simulink model "KR6_dyn_lib"  (R2018a)
settings: Solver=VariableStepAuto  StartTime=0.0  StopTime=10.0  RelTol=1e-3
(part 2 of 2)

== matlab function KR6_dyn_lib/dynamics ==
  data: dq2 input; B output; dq3 input; dq4 input; dq5 input; dq6 input; dq7 input; g input; q2 input; q3 input; q4 input; q5 input; q6 input; Bm output; Phi output; Phim output; G output
function [B,Bm,Phi,Phim,G] = dynamics(dq2,dq3,dq4,dq5,dq6,dq7,g,q2,q3,q4,q5,q6)
%#codegen

%    This function was generated by the Symbolic Math Toolbox version 8.1.
%    27-May-2020 20:53:49

t2 = cos(q2);
t3 = sin(q2);
t4 = sin(q5);
t5 = cos(q3);
t6 = cos(q4);
t7 = sin(q3);
t8 = sin(q4);
t9 = cos(q5);
t10 = cos(q6);
t11 = sin(q6);
t12 = t7.*t8.*1.4164748e7;
t13 = t4.*t5.*t8.*1.79145e5;
t14 = t4.*t6.*t7.*1.79145e5;
t15 = t7.*t8.*t10.*1.42171e5;
t16 = t5.*t8.*t9.*t11.*1.42171e5;
t17 = t6.*t7.*t9.*t11.*1.42171e5;
t18 = t3.*5.02822e-2;
t19 = t3.*t4.*t11.*1.42171e-2;
t20 = t2.*t5.*t8.*1.4164748;
t21 = t2.*t6.*t7.*1.4164748;
t22 = t2.*t7.*t8.*2.37344e-1;
t23 = t2.*t4.*t5.*t6.*1.79145e-2;
t24 = t2.*t5.*t8.*t10.*1.42171e-2;
t25 = t2.*t6.*t7.*t10.*1.42171e-2;
t26 = t2.*t7.*t8.*t9.*4.582e-4;
t27 = t2.*t5.*t6.*t9.*t11.*1.42171e-2;
t28 = t2.*(-6.45733e-1)+t18+t19+t20+t21+t22+t23+t24+t25+t26+t27-t2.*t5.*4.812199-t3.*t4.*4.582e-4-t2.*t7.*6.51847e-2-t3.*t9.*1.79145e-2-t2.*t5.*t6.*2.37344e-1-t2.*t4.*t7.*t8.*1.79145e-2-t2.*t5.*t6.*t9.*4.582e-4-t2.*t7.*t8.*t9.*t11.*1.42171e-2;
t29 = q3.*2.0;
t30 = q5.*2.0;
t31 = cos(t29);
t32 = sin(t29);
t33 = sin(t30);
t34 = cos(t30);
t35 = q6.*2.0;
t36 = cos(t35);
t37 = q4.*2.0;
t38 = cos(t37);
t39 = sin(t37);
t40 = sin(t35);
t41 = t4.*t7.*t8.*1.0579838e-4;
t42 = t5.*t8.*t33.*1.2735850275e-3;
t43 = t6.*t7.*t33.*1.2735850275e-3;
t44 = t7.*t8.*t9.*4.62678618e-3;
t45 = t5.*t8.*t11.*t34.*2.384424e-5;
t46 = t6.*t7.*t11.*t34.*2.384424e-5;
t47 = t4.*t5.*t6.*t40.*4.14863515e-4;
t48 = t5.*t8.*t33.*t36.*2.074317575e-4;
t49 = t6.*t7.*t33.*t36.*2.074317575e-4;
t50 = t4.*t5.*t6.*t11.*5.1892415e-3;
t51 = t7.*t8.*t9.*t10.*2.384424e-5;
t52 = t4.*t5.*t8.*t11.*4.975985e-4;
t53 = t4.*t6.*t7.*t11.*4.975985e-4;
t54 = t10.^2;
t55 = t5.*6.51847e5;
t56 = t7.*4.812199e7;
t68 = t5.*t6.*1.4164748e7;
t69 = t5.*t8.*2.37344e6;
t70 = t6.*t7.*2.37344e6;
t71 = t5.*t6.*t10.*1.42171e5;
t72 = t5.*t8.*t9.*4.582e3;
t73 = t6.*t7.*t9.*4.582e3;
t57 = t12+t13+t14+t15+t16+t17+t55-t56-t68-t69-t70-t71-t72-t73;
t58 = t7.*1.21447802e-2;
t59 = t4.*t7.*t11.*4.4783865e-3;
t74 = t5.*t8.*t34.*1.64952e-6;
t75 = t6.*t7.*t34.*1.64952e-6;
t76 = t5.*t6.*t9.*4.62678618e-3;
t77 = t4.*t5.*t6.*1.0579838e-4;
t78 = t5.*t8.*t9.*6.270075e-4;
t79 = t6.*t7.*t9.*6.270075e-4;
t80 = t4.*t5.*t8.*1.6037e-5;
t81 = t4.*t6.*t7.*1.6037e-5;
t82 = t4.*t7.*t8.*t40.*4.14863515e-4;
t83 = t5.*t6.*t9.*t10.*2.384424e-5;
t84 = t4.*t7.*t8.*t11.*5.1892415e-3;
t60 = t5.*(-3.7807126e-4)+t41+t42+t43+t44+t45+t46+t47+t48+t49+t50+t51+t52+t53+t58+t59-t74-t75-t76-t77-t78-t79-t80-t81-t82-t83-t84-t4.*t7.*1.44333e-4-t7.*t9.*5.6430675e-3;
t61 = t9.^2;
t62 = t6.*7.476336e-2;
t63 = t9.*3.2074e-5;
t64 = t10.*1.0378483e-2;
t65 = t6.*t9.*1.44333e-4;
t66 = t54.*8.2972703e-4;
t67 = t4.*t9.*t11.*4.768848e-5;
t86 = t33.*1.64952e-6;
t87 = t4.*1.254015e-3;
t88 = t9.*t11.*9.95197e-4;
t89 = t61.*2.13230654e-3;
t90 = t54.*t61.*8.2972703e-4;
t85 = t8.*(-4.46189562e-1)+t62+t63+t64+t65+t66+t67-t86-t87-t88-t89-t90-t4.*t6.*5.6430675e-3-t8.*t10.*4.4783865e-3-t6.*t9.*t11.*4.4783865e-3+4.0306203851e-1;
t91 = t9.*4.62678618e-3;
t92 = t4.*1.0579838e-4;
t93 = t9.*t10.*2.384424e-5;
t94 = t9.*1.23472703e-3;
t95 = t9.*t10.*5.1892415e-3;
t96 = t4.*t11.*2.384424e-5;
t97 = t4.*t11.*5.0e-6;
t98 = t2.*t9.*4.582e-4;
t99 = t3.*t5.*t6.*t9.*1.79145e-2;
t100 = t3.*t4.*t5.*t6.*4.582e-4;
t101 = t3.*t4.*t7.*t8.*t11.*1.42171e-2;
t102 = t98+t99+t100+t101-t2.*t4.*1.79145e-2-t2.*t9.*t11.*1.42171e-2-t3.*t4.*t7.*t8.*4.582e-4-t3.*t7.*t8.*t9.*1.79145e-2-t3.*t4.*t5.*t6.*t11.*1.42171e-2;
t103 = t4.*4.478625e-4;
t104 = t4.*t5.*5.6430675e-3;
t105 = t9.*t11.*3.554275e-4;
t106 = t4.*t5.*t6.*6.270075e-4;
t107 = t5.*t8.*t9.*1.0579838e-4;
t108 = t6.*t7.*t9.*1.0579838e-4;
t109 = t5.*t9.*t11.*4.4783865e-3;
t110 = t7.*t8.*t9.*1.6037e-5;
t111 = t5.*t6.*t9.*t11.*4.975985e-4;
t112 = t4.*t8.*t11.*4.4783865e-3;
t114 = t4.*t11.*5.1892415e-3;
t115 = t4.*t10.*t11.*8.2972703e-4;
t113 = t91+t92+t93+t112-t114-t115-t4.*t8.*1.44333e-4-t8.*t9.*5.6430675e-3;
t116 = t3.*t5.*t6.*t9.*t10.*1.42171e-2;
t117 = t116-t2.*t4.*t10.*1.42171e-2-t3.*t5.*t8.*t11.*1.42171e-2-t3.*t6.*t7.*t11.*1.42171e-2-t3.*t7.*t8.*t9.*t10.*1.42171e-2;
t118 = t4.*t10.*3.554275e-4;
t119 = t4.*t5.*t10.*4.4783865e-3;
t120 = t7.*t8.*t10.*2.384424e-5;
t121 = t4.*t5.*t6.*t10.*4.975985e-4;
t122 = t5.*t8.*t9.*t11.*2.384424e-5;
t123 = t6.*t7.*t9.*t11.*2.384424e-5;
t124 = t118+t119+t120+t121+t122+t123-t4.*t5.*t8.*1.23472703e-3-t4.*t6.*t7.*1.23472703e-3-t5.*t6.*t10.*2.384424e-5-t4.*t5.*t8.*t10.*5.1892415e-3-t4.*t6.*t7.*t10.*5.1892415e-3-t4.*t7.*t8.*t10.*4.975985e-4;
t126 = t11.*4.975985e-4;
t125 = t94+t95+t96-t126-t6.*t11.*4.4783865e-3-t8.*t9.*t10.*4.4783865e-3;
t127 = t10.*2.384424e-5;
t128 = q3+q4;
t129 = t10.*5.0e-6;
t130 = sin(t128);
t131 = cos(t128);
t132 = t4.^2;
t133 = t9-t4.*t11;
t134 = t11.^2;
B = reshape([8.714e1,t28,t3.*t57.*(-1.0e-7),t3.*(t12+t13+t14+t15+t16+t17-t68-t69-t70-t71-t72-t73).*(-1.0e-7),t102,t117,0.0,t28,t4.*(-6.270075e-4)+t5.*2.4060995e-1+t7.*3.259235e-3-t8.*4.46189562e-1+t9.*1.6037e-5+t10.*5.1892415e-3+t31.*7.03321055045e-1+t32.*1.00391957e-2+t33.*8.2476e-7+t34.*6.3679251375e-4-t36.*1.0371587875e-4+t62+t65-t4.*t6.*5.6430675e-3+t5.*t6.*1.18672e-2-t5.*t8.*7.082374e-2-t6.*t7.*7.082374e-2-t7.*t8.*1.18672e-2-t8.*t10.*4.4783865e-3-t9.*t11.*4.975985e-4+t6.*t31.*7.476336e-2-t6.*t32.*4.46189562e-1-t8.*t31.*4.46189562e-1-t8.*t32.*7.476336e-2-t11.*t33.*1.192212e-5-t31.*t38.*1.8083421453625e-1-t31.*t39.*4.99715694e-2-t32.*t38.*4.99715694e-2+t34.*t36.*1.0371587875e-4+t32.*t39.*1.8083421453625e-1-t4.*t5.*t6.*8.95725e-4+t4.*t7.*t8.*8.95725e-4+t5.*t6.*t9.*2.291e-5-t5.*t8.*t10.*7.10855e-4-t6.*t7.*t10.*7.10855e-4-t7.*t8.*t9.*2.291e-5-t6.*t9.*t11.*4.4783865e-3-t4.*t6.*t31.*5.6430675e-3+t4.*t8.*t32.*5.6430675e-3+t6.*t9.*t31.*1.44333e-4-t6.*t10.*t32.*4.4783865e-3-t8.*t9.*t32.*1.44333e-4-t8.*t10.*t31.*4.4783865e-3-t4.*t31.*t38.*6.270075e-4+t4.*t31.*t39.*4.62678618e-3+t4.*t32.*t38.*4.62678618e-3+t4.*t32.*t39.*6.270075e-4+t9.*t31.*t38.*1.6037e-5-t9.*t31.*t39.*1.0579838e-4-t9.*t32.*t38.*1.0579838e-4-t10.*t31.*t38.*5.1892415e-3-t9.*t32.*t39.*1.6037e-5-t10.*t31.*t39.*4.975985e-4-t10.*t32.*t38.*4.975985e-4+t10.*t32.*t39.*5.1892415e-3-t31.*t33.*t38.*8.2476e-7-t31.*t34.*t38.*6.3679251375e-4+t32.*t33.*t39.*8.2476e-7-t31.*t36.*t38.*3.1114763625e-4+t32.*t34.*t39.*6.3679251375e-4+t32.*t36.*t39.*3.1114763625e-4-t5.*t6.*t9.*t11.*7.10855e-4+t7.*t8.*t9.*t11.*7.10855e-4-t6.*t9.*t11.*t31.*4.4783865e-3+t8.*t9.*t11.*t32.*4.4783865e-3+t4.*t10.*t31.*t39.*2.384424e-5+t4.*t10.*t32.*t38.*2.384424e-5-t9.*t11.*t31.*t38.*4.975985e-4+t9.*t11.*t31.*t39.*5.1892415e-3+t9.*t11.*t32.*t38.*5.1892415e-3+t9.*t11.*t32.*t39.*4.975985e-4+t11.*t31.*t33.*t38.*1.192212e-5-t11.*t32.*t33.*t39.*1.192212e-5+t9.*t31.*t39.*t40.*4.14863515e-4+t9.*t32.*t38.*t40.*4.14863515e-4-t31.*t34.*t36.*t38.*1.0371587875e-4+t32.*t34.*t36.*t39.*1.0371587875e-4+1.08912681817625,t60,t41+t42+t43+t44+t45+t46+t47+t48+t49+t50+t51+t52+t53-t74-t75-t76-t77-t78-t79-t80-t81-t82-t83-t84,t9.*(-1.1455e-5)+t103+t104+t105+t106+t107+t108+t109+t110+t111-t5.*t6.*1.0581988725e-2-t5.*t9.*1.44333e-4+t7.*t8.*1.0581988725e-2-t4.*t5.*t8.*4.62678618e-3-t4.*t6.*t7.*4.62678618e-3-t4.*t7.*t8.*6.270075e-4-t5.*t6.*t9.*1.6037e-5+t5.*t6.*t36.*4.14863515e-4-t7.*t8.*t36.*4.14863515e-4-t4.*t5.*t8.*t10.*2.384424e-5-t4.*t6.*t7.*t10.*2.384424e-5-t5.*t8.*t9.*t11.*5.1892415e-3-t6.*t7.*t9.*t11.*5.1892415e-3-t7.*t8.*t9.*t11.*4.975985e-4-t5.*t8.*t9.*t40.*4.14863515e-4-t6.*t7.*t9.*t40.*4.14863515e-4,t124,t10.*t131.*(-5.0e-6)+t9.*t11.*t130.*5.0e-6,t3.*t57.*(-1.0e-7),t60,t4.*(-1.254015e-3)+t6.*1.4952672e-1-t8.*8.92379124e-1-t33.*1.64952e-6-t61.*2.13230654e-3+t63+t64+t66+t67-t4.*t6.*1.1286135e-2+t6.*t9.*2.88666e-4-t8.*t10.*8.956773e-3-t9.*t11.*9.95197e-4-t54.*t61.*8.2972703e-4-t6.*t9.*t11.*8.956773e-3+1.84829510642,t85,t113,t125,t97,t3.*(t12+t13+t14+t15+t16+t17-t5.*t6.*1.4164748e7-t5.*t8.*2.37344e6-t6.*t7.*2.37344e6-t5.*t6.*t10.*1.42171e5-t5.*t8.*t9.*4.582e3-t6.*t7.*t9.*4.582e3).*(-1.0e-7),t41+t42+t43+t44+t45+t46+t47+t48+t49+t50+t51+t52+t53-t4.*t5.*t6.*1.0579838e-4-t4.*t5.*t8.*1.6037e-5-t4.*t6.*t7.*1.6037e-5-t5.*t6.*t9.*4.62678618e-3-t5.*t8.*t9.*6.270075e-4-t6.*t7.*t9.*6.270075e-4-t5.*t8.*t34.*1.64952e-6-t6.*t7.*t34.*1.64952e-6-t4.*t7.*t8.*t11.*5.1892415e-3-t5.*t6.*t9.*t10.*2.384424e-5-t4.*t7.*t8.*t40.*4.14863515e-4,t85,t63+t64+t66+t67-t86-t87-t88-t89-t90+4.0306203851e-1,t91+t92+t93-t114-t115,t94+t95+t96-t126,t97,t102,t9.*(-1.1455e-5)+t103+t104+t105+t106+t107+t108+t109+t110+t111-t5.*t6.*1.099685224e-2-t5.*t9.*1.44333e-4+t7.*t8.*1.099685224e-2-t4.*t5.*t8.*4.62678618e-3-t4.*t6.*t7.*4.62678618e-3-t4.*t7.*t8.*6.270075e-4-t5.*t6.*t9.*1.6037e-5+t5.*t6.*t54.*8.2972703e-4-t7.*t8.*t54.*8.2972703e-4-t4.*t5.*t8.*t10.*2.384424e-5-t4.*t6.*t7.*t10.*2.384424e-5-t5.*t8.*t9.*t11.*5.1892415e-3-t6.*t7.*t9.*t11.*5.1892415e-3-t7.*t8.*t9.*t11.*4.975985e-4-t5.*t8.*t9.*t10.*t11.*8.2972703e-4-t6.*t7.*t9.*t10.*t11.*8.2972703e-4,t113,t91+t92+t93-t4.*t11.*5.1892415e-3-t4.*t10.*t11.*8.2972703e-4,t134.*8.2972703e-4+1.016712521e-2,t127,t129,t117,t124,t125,t11.*(-4.975985e-4)+t94+t95+t96,t127,1.23472703e-3,0.0,0.0,-t5.*(t6.*t10.*5.0e-6-t8.*t9.*t11.*5.0e-6)+t7.*(t8.*t10.*5.0e-6+t6.*t9.*t11.*5.0e-6),t97,t97,t129,0.0,5.0e-6],[7,7]);
if nargout > 1
    Bm = reshape([2.1e1./1.0e1,0.0,0.0,0.0,0.0,0.0,0.0,0.0,2.1e1./1.0e1,t2.*(-2.1e1./1.0e3),0.0,t8.*t130.*(2.1e1./1.0e3),t9.*t131.*(2.1e1./1.0e3)-t33.*t130.*1.05e-2,t11.*(t11.*t131.*(2.1e1./1.0e3)+t9.*t10.*t130.*(2.1e1./1.0e3))+t4.*t10.*t130.*(2.1e1./1.0e3),0.0,t2.*(-2.1e1./1.0e3),2.1e1./1.0e1,2.1e1./1.0e3,t6.*(-2.1e1./1.0e3),t132.*(-2.1e1./1.0e3),t10.*t133.*(-2.1e1./1.0e3),0.0,0.0,2.1e1./1.0e3,2.1e1./1.0e1,t6.*(-2.1e1./1.0e3),t132.*(-2.1e1./1.0e3),t10.*t133.*(-2.1e1./1.0e3),0.0,0.0,0.0,t6.*(-2.1e1./1.0e3),2.1e1./1.0e1,t9.*(-2.1e1./1.0e3),t134.*(-2.1e1./1.0e3),0.0,0.0,0.0,0.0,t9.*(-2.1e1./1.0e3),2.1e1./1.0e1,t10.*(-2.1e1./1.0e3),0.0,0.0,0.0,0.0,0.0,t10.*(-2.1e1./1.0e3),2.1e1./1.0e1],[7,7]);
end
if nargout > 2
    t135 = dq2.^2;
    t136 = dq5.^2;
    t137 = dq3.^2;
    t138 = dq4.^2;
    t139 = dq6.^2;
    t140 = t9.*t136.*1.0579838e-4;
    t141 = dq3.*dq5.*t33.*2.547170055e-3;
    t142 = dq4.*dq5.*t33.*2.547170055e-3;
    t143 = t31.*t38.*t135.*4.99715694e-2;
    t144 = t5.*t6.*t135.*3.541187e-2;
    t145 = t5.*t8.*t135.*5.9336e-3;
    t146 = t6.*t7.*t135.*5.9336e-3;
    t147 = t4.*t10.*t139.*2.384424e-5;
    t148 = dq3.*dq5.*t11.*t34.*4.768848e-5;
    t149 = dq3.*dq6.*t10.*t33.*2.384424e-5;
    t150 = dq4.*dq5.*t11.*t34.*4.768848e-5;
    t151 = dq4.*dq6.*t10.*t33.*2.384424e-5;
    t152 = t9.*t31.*t38.*t135.*1.0579838e-4;
    t153 = t10.*t31.*t38.*t135.*4.975985e-4;
    t154 = t9.*t31.*t39.*t135.*1.6037e-5;
    t155 = t9.*t32.*t38.*t135.*1.6037e-5;
    t156 = t4.*t32.*t39.*t135.*4.62678618e-3;
    t157 = dq3.*dq5.*t33.*t36.*4.14863515e-4;
    t158 = dq3.*dq6.*t34.*t40.*4.14863515e-4;
    t159 = dq4.*dq5.*t33.*t36.*4.14863515e-4;
    t160 = dq4.*dq6.*t34.*t40.*4.14863515e-4;
    t161 = t5.*t6.*t10.*t135.*3.554275e-4;
    t162 = t5.*t8.*t9.*t135.*1.1455e-5;
    t163 = t6.*t7.*t9.*t135.*1.1455e-5;
    t164 = dq5.*dq7.*t9.*t11.*5.0e-6;
    t165 = dq6.*dq7.*t4.*t10.*5.0e-6;
    t166 = dq3.*dq5.*t4.*t11.*9.95197e-4;
    t167 = dq4.*dq5.*t4.*t11.*9.95197e-4;
    t168 = dq2.*dq5.*t5.*t8.*t34.*2.547170055e-3;
    t169 = dq2.*dq5.*t6.*t7.*t34.*2.547170055e-3;
    t170 = dq2.*dq5.*t5.*t8.*t36.*4.14863515e-4;
    t171 = dq2.*dq5.*t6.*t7.*t36.*4.14863515e-4;
    t172 = dq2.*dq5.*t5.*t8.*t33.*3.29904e-6;
    t173 = dq2.*dq5.*t6.*t7.*t33.*3.29904e-6;
    t174 = t9.*t11.*t32.*t39.*t135.*5.1892415e-3;
    t175 = t4.*t10.*t32.*t39.*t135.*2.384424e-5;
    t176 = dq2.*dq5.*t4.*t5.*t6.*9.25357236e-3;
    t177 = dq2.*dq6.*t4.*t5.*t6.*1.23472703e-3;
    t178 = t11.*t31.*t33.*t39.*t135.*1.192212e-5;
    t179 = t11.*t32.*t33.*t38.*t135.*1.192212e-5;
    t180 = t9.*t32.*t39.*t40.*t135.*4.14863515e-4;
    t181 = dq2.*dq5.*t4.*t5.*t8.*1.254015e-3;
    t182 = dq2.*dq5.*t4.*t6.*t7.*1.254015e-3;
    t183 = dq2.*dq5.*t7.*t8.*t9.*2.1159676e-4;
    t184 = dq2.*dq5.*t5.*t8.*t34.*t36.*4.14863515e-4;
    t185 = dq2.*dq5.*t6.*t7.*t34.*t36.*4.14863515e-4;
    t186 = dq2.*dq5.*t5.*t6.*t9.*t11.*1.0378483e-2;
    t187 = dq2.*dq5.*t4.*t5.*t6.*t10.*4.768848e-5;
    t188 = dq2.*dq6.*t4.*t5.*t6.*t10.*1.0378483e-2;
    t189 = dq2.*dq5.*t5.*t8.*t9.*t11.*9.95197e-4;
    t190 = dq2.*dq5.*t6.*t7.*t9.*t11.*9.95197e-4;
    t191 = dq2.*dq6.*t4.*t5.*t8.*t10.*9.95197e-4;
    t192 = dq2.*dq6.*t4.*t6.*t7.*t10.*9.95197e-4;
    t193 = dq2.*dq7.*t7.*t8.*t9.*t11.*5.0e-6;
    t194 = dq2.*dq5.*t5.*t6.*t9.*t40.*8.2972703e-4;
    t195 = dq2.*dq6.*t5.*t8.*t10.*t34.*2.384424e-5;
    t196 = dq2.*dq6.*t6.*t7.*t10.*t34.*2.384424e-5;
    t197 = dq2.*dq6.*t4.*t5.*t6.*t36.*8.2972703e-4;
    Phi = [t2.*t135.*5.02822e-2+t3.*t135.*6.45733e-1-t2.*t4.*t135.*4.582e-4-t2.*t4.*t136.*4.582e-4+t3.*t5.*t135.*4.812199+t3.*t5.*t137.*4.812199+t3.*t7.*t135.*6.51847e-2-t2.*t9.*t135.*1.79145e-2-t2.*t9.*t136.*1.79145e-2+t3.*t7.*t137.*6.51847e-2-dq2.*dq3.*t2.*t5.*1.303694e-1+dq2.*dq3.*t2.*t7.*9.624398+dq2.*dq5.*t3.*t4.*3.5829e-2-dq2.*dq5.*t3.*t9.*9.164e-4+t3.*t5.*t6.*t135.*2.37344e-1+t3.*t5.*t6.*t137.*2.37344e-1-t3.*t5.*t8.*t135.*1.4164748-t3.*t6.*t7.*t135.*1.4164748+t2.*t4.*t11.*t135.*1.42171e-2+t3.*t5.*t6.*t138.*2.37344e-1+t2.*t4.*t11.*t136.*1.42171e-2-t3.*t5.*t8.*t137.*1.4164748-t3.*t6.*t7.*t137.*1.4164748-t3.*t7.*t8.*t135.*2.37344e-1-t3.*t5.*t8.*t138.*1.4164748-t3.*t6.*t7.*t138.*1.4164748-t3.*t7.*t8.*t137.*2.37344e-1+t2.*t4.*t11.*t139.*1.42171e-2-t3.*t7.*t8.*t138.*2.37344e-1+dq2.*dq3.*t2.*t5.*t6.*2.8329496+dq2.*dq4.*t2.*t5.*t6.*2.8329496+dq2.*dq3.*t2.*t5.*t8.*4.74688e-1+dq2.*dq3.*t2.*t6.*t7.*4.74688e-1+dq2.*dq4.*t2.*t5.*t8.*4.74688e-1+dq2.*dq4.*t2.*t6.*t7.*4.74688e-1+dq3.*dq4.*t3.*t5.*t6.*4.74688e-1-dq2.*dq3.*t2.*t7.*t8.*2.8329496-dq2.*dq4.*t2.*t7.*t8.*2.8329496-dq3.*dq4.*t3.*t5.*t8.*2.8329496-dq3.*dq4.*t3.*t6.*t7.*2.8329496+dq2.*dq6.*t3.*t4.*t10.*2.84342e-2-dq3.*dq4.*t3.*t7.*t8.*4.74688e-1+dq2.*dq5.*t3.*t9.*t11.*2.84342e-2-dq5.*dq6.*t2.*t9.*t10.*2.84342e-2-t3.*t4.*t5.*t6.*t135.*1.79145e-2-t3.*t4.*t5.*t6.*t136.*1.79145e-2-t3.*t4.*t5.*t6.*t137.*1.79145e-2-t3.*t4.*t5.*t6.*t138.*1.79145e-2+t3.*t4.*t7.*t8.*t135.*1.79145e-2+t3.*t4.*t7.*t8.*t136.*1.79145e-2+t3.*t5.*t6.*t9.*t135.*4.582e-4+t3.*t4.*t7.*t8.*t137.*1.79145e-2+t3.*t5.*t6.*t9.*t136.*4.582e-4+t3.*t4.*t7.*t8.*t138.*1.79145e-2+t3.*t5.*t6.*t9.*t137.*4.582e-4+t3.*t5.*t6.*t9.*t138.*4.582e-4-t3.*t5.*t8.*t10.*t135.*1.42171e-2-t3.*t6.*t7.*t10.*t135.*1.42171e-2-t3.*t7.*t8.*t9.*t135.*4.582e-4-t3.*t5.*t8.*t10.*t137.*1.42171e-2-t3.*t6.*t7.*t10.*t137.*1.42171e-2-t3.*t7.*t8.*t9.*t136.*4.582e-4-t3.*t5.*t8.*t10.*t138.*1.42171e-2-t3.*t6.*t7.*t10.*t138.*1.42171e-2-t3.*t7.*t8.*t9.*t137.*4.582e-4-t3.*t5.*t8.*t10.*t139.*1.42171e-2-t3.*t6.*t7.*t10.*t139.*1.42171e-2-t3.*t7.*t8.*t9.*t138.*4.582e-4-t3.*t5.*t6.*t9.*t11.*t135.*1.42171e-2-t3.*t5.*t6.*t9.*t11.*t136.*1.42171e-2-t3.*t5.*t6.*t9.*t11.*t137.*1.42171e-2-t3.*t5.*t6.*t9.*t11.*t138.*1.42171e-2-t3.*t5.*t6.*t9.*t11.*t139.*1.42171e-2+t3.*t7.*t8.*t9.*t11.*t135.*1.42171e-2+t3.*t7.*t8.*t9.*t11.*t136.*1.42171e-2+t3.*t7.*t8.*t9.*t11.*t137.*1.42171e-2+t3.*t7.*t8.*t9.*t11.*t138.*1.42171e-2+t3.*t7.*t8.*t9.*t11.*t139.*1.42171e-2-dq2.*dq3.*t2.*t4.*t5.*t8.*3.5829e-2-dq2.*dq3.*t2.*t4.*t6.*t7.*3.5829e-2+dq2.*dq5.*t2.*t4.*t5.*t6.*9.164e-4-dq2.*dq4.*t2.*t4.*t5.*t8.*3.5829e-2-dq2.*dq4.*t2.*t4.*t6.*t7.*3.5829e-2-dq3.*dq4.*t3.*t4.*t5.*t6.*3.5829e-2+dq2.*dq3.*t2.*t5.*t6.*t10.*2.84342e-2-dq2.*dq5.*t2.*t4.*t7.*t8.*9.164e-4-dq3.*dq5.*t3.*t4.*t5.*t8.*9.164e-4-dq3.*dq5.*t3.*t4.*t6.*t7.*9.164e-4+dq2.*dq3.*t2.*t5.*t8.*t9.*9.164e-4+dq2.*dq3.*t2.*t6.*t7.*t9.*9.164e-4+dq2.*dq4.*t2.*t5.*t6.*t10.*2.84342e-2+dq2.*dq5.*t2.*t5.*t6.*t9.*3.5829e-2+dq3.*dq4.*t3.*t4.*t7.*t8.*3.5829e-2-dq4.*dq5.*t3.*t4.*t5.*t8.*9.164e-4-dq4.*dq5.*t3.*t4.*t6.*t7.*9.164e-4+dq2.*dq4.*t2.*t5.*t8.*t9.*9.164e-4+dq2.*dq4.*t2.*t6.*t7.*t9.*9.164e-4+dq3.*dq4.*t3.*t5.*t6.*t9.*9.164e-4-dq2.*dq3.*t2.*t7.*t8.*t10.*2.84342e-2-dq2.*dq4.*t2.*t7.*t8.*t10.*2.84342e-2-dq2.*dq5.*t2.*t7.*t8.*t9.*3.5829e-2-dq3.*dq4.*t3.*t5.*t8.*t10.*2.84342e-2-dq3.*dq4.*t3.*t6.*t7.*t10.*2.84342e-2-dq3.*dq5.*t3.*t5.*t8.*t9.*3.5829e-2-dq3.*dq5.*t3.*t6.*t7.*t9.*3.5829e-2-dq2.*dq6.*t2.*t5.*t8.*t11.*2.84342e-2-dq2.*dq6.*t2.*t6.*t7.*t11.*2.84342e-2-dq3.*dq4.*t3.*t7.*t8.*t9.*9.164e-4-dq3.*dq6.*t3.*t5.*t6.*t11.*2.84342e-2-dq4.*dq5.*t3.*t5.*t8.*t9.*3.5829e-2-dq4.*dq5.*t3.*t6.*t7.*t9.*3.5829e-2-dq4.*dq6.*t3.*t5.*t6.*t11.*2.84342e-2+dq3.*dq6.*t3.*t7.*t8.*t11.*2.84342e-2+dq4.*dq6.*t3.*t7.*t8.*t11.*2.84342e-2-dq2.*dq5.*t2.*t4.*t5.*t6.*t11.*2.84342e-2+dq2.*dq5.*t2.*t4.*t7.*t8.*t11.*2.84342e-2+dq3.*dq5.*t3.*t4.*t5.*t8.*t11.*2.84342e-2+dq3.*dq5.*t3.*t4.*t6.*t7.*t11.*2.84342e-2-dq5.*dq6.*t3.*t4.*t5.*t6.*t10.*2.84342e-2-dq2.*dq3.*t2.*t5.*t8.*t9.*t11.*2.84342e-2-dq2.*dq3.*t2.*t6.*t7.*t9.*t11.*2.84342e-2+dq2.*dq6.*t2.*t5.*t6.*t9.*t10.*2.84342e-2+dq4.*dq5.*t3.*t4.*t5.*t8.*t11.*2.84342e-2+dq4.*dq5.*t3.*t4.*t6.*t7.*t11.*2.84342e-2-dq2.*dq4.*t2.*t5.*t8.*t9.*t11.*2.84342e-2-dq2.*dq4.*t2.*t6.*t7.*t9.*t11.*2.84342e-2-dq3.*dq4.*t3.*t5.*t6.*t9.*t11.*2.84342e-2+dq5.*dq6.*t3.*t4.*t7.*t8.*t10.*2.84342e-2-dq2.*dq6.*t2.*t7.*t8.*t9.*t10.*2.84342e-2-dq3.*dq6.*t3.*t5.*t8.*t9.*t10.*2.84342e-2-dq3.*dq6.*t3.*t6.*t7.*t9.*t10.*2.84342e-2+dq3.*dq4.*t3.*t7.*t8.*t9.*t11.*2.84342e-2-dq4.*dq6.*t3.*t5.*t8.*t9.*t10.*2.84342e-2-dq4.*dq6.*t3.*t6.*t7.*t9.*t10.*2.84342e-2;t4.*t136.*1.1455e-5+t5.*t137.*1.21447802e-2+t7.*t137.*3.7807126e-4+t9.*t136.*4.478625e-4+dq2.*dq3.*t5.*3.259235e-3-dq2.*dq5.*t4.*1.6037e-5-dq2.*dq3.*t7.*2.4060995e-1-dq2.*dq4.*t6.*4.46189562e-1-dq2.*dq4.*t8.*7.476336e-2-dq2.*dq5.*t9.*6.270075e-4-dq2.*dq6.*t11.*5.1892415e-3+dq2.*dq3.*t31.*2.00783914e-2-dq2.*dq3.*t32.*1.40664211009-dq2.*dq5.*t33.*1.2735850275e-3+dq2.*dq5.*t34.*1.64952e-6+dq2.*dq6.*t40.*2.074317575e-4+t4.*t5.*t136.*1.44333e-4-t4.*t5.*t137.*1.44333e-4+t5.*t9.*t136.*5.6430675e-3-t4.*t11.*t136.*3.554275e-4-t5.*t9.*t137.*5.6430675e-3-t4.*t11.*t139.*3.554275e-4-dq2.*dq3.*t5.*t6.*7.082374e-2-dq2.*dq4.*t5.*t6.*7.082374e-2-dq2.*dq5.*t4.*t6.*1.44333e-4-dq2.*dq3.*t5.*t8.*1.18672e-2-dq2.*dq3.*t6.*t7.*1.18672e-2+dq2.*dq4.*t4.*t8.*5.6430675e-3-dq2.*dq4.*t5.*t8.*1.18672e-2-dq2.*dq4.*t6.*t7.*1.18672e-2+dq2.*dq3.*t7.*t8.*7.082374e-2+dq2.*dq4.*t7.*t8.*7.082374e-2+dq3.*dq5.*t5.*t8.*1.0581988725e-2+dq3.*dq5.*t6.*t7.*1.0581988725e-2-dq2.*dq4.*t6.*t10.*4.4783865e-3+dq2.*dq5.*t4.*t11.*4.975985e-4-dq2.*dq5.*t6.*t9.*5.6430675e-3+dq4.*dq5.*t5.*t8.*1.0581988725e-2+dq4.*dq5.*t6.*t7.*1.0581988725e-2-dq2.*dq4.*t8.*t9.*1.44333e-4+dq2.*dq6.*t8.*t11.*4.4783865e-3-dq2.*dq6.*t9.*t10.*4.975985e-4+dq5.*dq6.*t9.*t10.*7.10855e-4-dq2.*dq3.*t6.*t31.*8.92379124e-1-dq2.*dq3.*t6.*t32.*1.4952672e-1-dq2.*dq4.*t6.*t31.*4.46189562e-1-dq2.*dq3.*t8.*t31.*1.4952672e-1-dq2.*dq4.*t6.*t32.*7.476336e-2+dq2.*dq3.*t8.*t32.*8.92379124e-1-dq2.*dq4.*t8.*t31.*7.476336e-2+dq2.*dq4.*t8.*t32.*4.46189562e-1-dq2.*dq6.*t10.*t33.*1.192212e-5-dq2.*dq5.*t11.*t34.*2.384424e-5-dq2.*dq3.*t31.*t38.*9.99431388e-2+dq2.*dq3.*t31.*t39.*3.616684290725e-1+dq2.*dq3.*t32.*t38.*3.616684290725e-1-dq2.*dq4.*t31.*t38.*9.99431388e-2+dq2.*dq3.*t32.*t39.*9.99431388e-2+dq2.*dq4.*t31.*t39.*3.616684290725e-1+dq2.*dq4.*t32.*t38.*3.616684290725e-1-dq2.*dq5.*t33.*t36.*2.074317575e-4+dq2.*dq4.*t32.*t39.*9.99431388e-2-dq2.*dq6.*t34.*t40.*2.074317575e-4+t4.*t5.*t6.*t136.*1.6037e-5-t4.*t5.*t6.*t137.*1.6037e-5-t4.*t5.*t6.*t138.*1.6037e-5-t4.*t5.*t8.*t136.*1.0579838e-4-t4.*t6.*t7.*t136.*1.0579838e-4+t4.*t5.*t8.*t137.*1.0579838e-4+t4.*t6.*t7.*t137.*1.0579838e-4+t4.*t5.*t8.*t138.*1.0579838e-4+t4.*t6.*t7.*t138.*1.0579838e-4-t4.*t7.*t8.*t136.*1.6037e-5-t4.*t5.*t11.*t136.*4.4783865e-3+t4.*t7.*t8.*t137.*1.6037e-5+t5.*t6.*t9.*t136.*6.270075e-4+t4.*t5.*t11.*t137.*4.4783865e-3+t4.*t7.*t8.*t138.*1.6037e-5-t5.*t6.*t9.*t137.*6.270075e-4-t5.*t6.*t9.*t138.*6.270075e-4-t5.*t8.*t9.*t136.*4.62678618e-3-t6.*t7.*t9.*t136.*4.62678618e-3-t4.*t5.*t11.*t139.*4.4783865e-3+t5.*t8.*t9.*t137.*4.62678618e-3+t6.*t7.*t9.*t137.*4.62678618e-3+t5.*t8.*t9.*t138.*4.62678618e-3+t6.*t7.*t9.*t138.*4.62678618e-3-t7.*t8.*t9.*t136.*6.270075e-4+t5.*t6.*t11.*t139.*2.384424e-5+t7.*t8.*t9.*t137.*6.270075e-4+t7.*t8.*t9.*t138.*6.270075e-4-t7.*t8.*t11.*t139.*2.384424e-5+t5.*t6.*t33.*t137.*1.2735850275e-3+t5.*t6.*t33.*t138.*1.2735850275e-3-t5.*t6.*t34.*t137.*1.64952e-6-t5.*t6.*t34.*t138.*1.64952e-6-t7.*t8.*t33.*t137.*1.2735850275e-3-t7.*t8.*t33.*t138.*1.2735850275e-3+t7.*t8.*t34.*t137.*1.64952e-6+t7.*t8.*t34.*t138.*1.64952e-6+dq2.*dq3.*t4.*t5.*t8.*8.95725e-4+dq2.*dq3.*t4.*t6.*t7.*8.95725e-4-dq2.*dq5.*t4.*t5.*t6.*2.291e-5-dq3.*dq4.*t4.*t5.*t6.*3.2074e-5+dq2.*dq4.*t4.*t5.*t8.*8.95725e-4+dq2.*dq4.*t4.*t6.*t7.*8.95725e-4+dq3.*dq4.*t4.*t5.*t8.*2.1159676e-4+dq3.*dq4.*t4.*t6.*t7.*2.1159676e-4-dq3.*dq6.*t4.*t5.*t6.*1.23472703e-3-dq4.*dq6.*t4.*t5.*t6.*1.23472703e-3-dq2.*dq3.*t5.*t6.*t10.*7.10855e-4+dq2.*dq5.*t4.*t7.*t8.*2.291e-5+dq3.*dq4.*t4.*t7.*t8.*3.2074e-5-dq2.*dq3.*t5.*t8.*t9.*2.291e-5-dq2.*dq3.*t6.*t7.*t9.*2.291e-5-dq2.*dq4.*t5.*t6.*t10.*7.10855e-4-dq2.*dq5.*t5.*t6.*t9.*8.95725e-4-dq3.*dq4.*t5.*t6.*t9.*1.254015e-3-dq2.*dq4.*t5.*t8.*t9.*2.291e-5-dq2.*dq4.*t6.*t7.*t9.*2.291e-5+dq2.*dq5.*t4.*t6.*t11.*4.4783865e-3+dq3.*dq6.*t4.*t7.*t8.*1.23472703e-3+dq3.*dq4.*t5.*t8.*t9.*9.25357236e-3+dq3.*dq4.*t6.*t7.*t9.*9.25357236e-3+dq4.*dq6.*t4.*t7.*t8.*1.23472703e-3+dq2.*dq3.*t7.*t8.*t10.*7.10855e-4+dq2.*dq4.*t7.*t8.*t10.*7.10855e-4+dq2.*dq5.*t7.*t8.*t9.*8.95725e-4+dq3.*dq4.*t7.*t8.*t9.*1.254015e-3+dq2.*dq6.*t5.*t8.*t11.*7.10855e-4+dq2.*dq6.*t6.*t7.*t11.*7.10855e-4+dq3.*dq6.*t5.*t8.*t10.*2.384424e-5+dq3.*dq6.*t6.*t7.*t10.*2.384424e-5-dq2.*dq6.*t6.*t9.*t10.*4.4783865e-3+dq3.*dq7.*t5.*t8.*t10.*5.0e-6+dq3.*dq7.*t6.*t7.*t10.*5.0e-6+dq4.*dq6.*t5.*t8.*t10.*2.384424e-5+dq4.*dq6.*t6.*t7.*t10.*2.384424e-5-dq5.*dq6.*t5.*t8.*t9.*1.23472703e-3-dq5.*dq6.*t6.*t7.*t9.*1.23472703e-3+dq2.*dq4.*t8.*t9.*t11.*4.4783865e-3+dq4.*dq7.*t5.*t8.*t10.*5.0e-6+dq4.*dq7.*t6.*t7.*t10.*5.0e-6+dq5.*dq6.*t5.*t9.*t10.*8.956773e-3+dq6.*dq7.*t5.*t6.*t11.*5.0e-6-dq6.*dq7.*t7.*t8.*t11.*5.0e-6+dq2.*dq3.*t4.*t6.*t32.*1.1286135e-2+dq2.*dq3.*t4.*t8.*t31.*1.1286135e-2+dq2.*dq4.*t4.*t6.*t32.*5.6430675e-3-dq2.*dq5.*t4.*t6.*t31.*1.44333e-4+dq2.*dq4.*t4.*t8.*t31.*5.6430675e-3+dq2.*dq5.*t4.*t8.*t32.*1.44333e-4+dq3.*dq4.*t5.*t6.*t33.*2.547170055e-3-dq2.*dq3.*t6.*t9.*t32.*2.88666e-4-dq2.*dq3.*t6.*t10.*t31.*8.956773e-3-dq3.*dq4.*t5.*t6.*t34.*3.29904e-6-dq2.*dq3.*t8.*t9.*t31.*2.88666e-4-dq2.*dq4.*t6.*t9.*t32.*1.44333e-4-dq2.*dq4.*t6.*t10.*t31.*4.4783865e-3-dq2.*dq5.*t6.*t9.*t31.*5.6430675e-3-dq2.*dq4.*t8.*t9.*t31.*1.44333e-4+dq3.*dq5.*t5.*t8.*t33.*3.29904e-6+dq3.*dq5.*t6.*t7.*t33.*3.29904e-6+dq2.*dq3.*t8.*t10.*t32.*8.956773e-3-dq3.*dq4.*t7.*t8.*t33.*2.547170055e-3+dq3.*dq5.*t5.*t8.*t34.*2.547170055e-3+dq3.*dq5.*t6.*t7.*t34.*2.547170055e-3+dq4.*dq5.*t5.*t8.*t33.*3.29904e-6+dq4.*dq5.*t6.*t7.*t33.*3.29904e-6+dq2.*dq4.*t8.*t10.*t32.*4.4783865e-3+dq2.*dq5.*t8.*t9.*t32.*5.6430675e-3+dq3.*dq4.*t7.*t8.*t34.*3.29904e-6+dq4.*dq5.*t5.*t8.*t34.*2.547170055e-3+dq4.*dq5.*t6.*t7.*t34.*2.547170055e-3+dq2.*dq6.*t6.*t11.*t32.*4.4783865e-3-dq3.*dq5.*t5.*t8.*t36.*4.14863515e-4-dq3.*dq5.*t6.*t7.*t36.*4.14863515e-4+dq2.*dq6.*t8.*t11.*t31.*4.4783865e-3-dq4.*dq5.*t5.*t8.*t36.*4.14863515e-4-dq4.*dq5.*t6.*t7.*t36.*4.14863515e-4-dq5.*dq6.*t5.*t6.*t40.*8.2972703e-4+dq5.*dq6.*t7.*t8.*t40.*8.2972703e-4+dq2.*dq3.*t4.*t31.*t38.*9.25357236e-3+dq2.*dq3.*t4.*t31.*t39.*1.254015e-3+dq2.*dq3.*t4.*t32.*t38.*1.254015e-3+dq2.*dq4.*t4.*t31.*t38.*9.25357236e-3-dq2.*dq3.*t4.*t32.*t39.*9.25357236e-3+dq2.*dq4.*t4.*t31.*t39.*1.254015e-3+dq2.*dq4.*t4.*t32.*t38.*1.254015e-3-dq2.*dq5.*t4.*t31.*t38.*1.6037e-5-dq2.*dq4.*t4.*t32.*t39.*9.25357236e-3+dq2.*dq5.*t4.*t31.*t39.*1.0579838e-4+dq2.*dq5.*t4.*t32.*t38.*1.0579838e-4+dq2.*dq5.*t4.*t32.*t39.*1.6037e-5-dq2.*dq3.*t9.*t31.*t38.*2.1159676e-4-dq2.*dq3.*t9.*t31.*t39.*3.2074e-5-dq2.*dq3.*t9.*t32.*t38.*3.2074e-5-dq2.*dq3.*t10.*t31.*t38.*9.95197e-4-dq2.*dq4.*t9.*t31.*t38.*2.1159676e-4+dq2.*dq3.*t9.*t32.*t39.*2.1159676e-4+dq2.*dq3.*t10.*t31.*t39.*1.0378483e-2+dq2.*dq3.*t10.*t32.*t38.*1.0378483e-2-dq2.*dq4.*t9.*t31.*t39.*3.2074e-5-dq2.*dq4.*t9.*t32.*t38.*3.2074e-5-dq2.*dq4.*t10.*t31.*t38.*9.95197e-4-dq2.*dq5.*t9.*t31.*t38.*6.270075e-4+dq2.*dq3.*t10.*t32.*t39.*9.95197e-4+dq2.*dq4.*t9.*t32.*t39.*2.1159676e-4+dq2.*dq4.*t10.*t31.*t39.*1.0378483e-2+dq2.*dq4.*t10.*t32.*t38.*1.0378483e-2+dq2.*dq5.*t9.*t31.*t39.*4.62678618e-3+dq2.*dq5.*t9.*t32.*t38.*4.62678618e-3+dq2.*dq4.*t10.*t32.*t39.*9.95197e-4+dq2.*dq5.*t9.*t32.*t39.*6.270075e-4+dq2.*dq6.*t11.*t31.*t38.*5.1892415e-3+dq2.*dq6.*t11.*t31.*t39.*4.975985e-4+dq2.*dq6.*t11.*t32.*t38.*4.975985e-4-dq2.*dq6.*t11.*t32.*t39.*5.1892415e-3+dq2.*dq3.*t31.*t33.*t39.*1.64952e-6+dq2.*dq3.*t32.*t33.*t38.*1.64952e-6+dq2.*dq3.*t31.*t34.*t39.*1.2735850275e-3+dq2.*dq3.*t32.*t34.*t38.*1.2735850275e-3+dq2.*dq4.*t31.*t33.*t39.*1.64952e-6+dq2.*dq4.*t32.*t33.*t38.*1.64952e-6+dq2.*dq5.*t31.*t33.*t38.*1.2735850275e-3+dq2.*dq4.*t31.*t34.*t39.*1.2735850275e-3+dq2.*dq4.*t32.*t34.*t38.*1.2735850275e-3-dq2.*dq5.*t31.*t34.*t38.*1.64952e-6+dq2.*dq3.*t31.*t36.*t39.*6.222952725e-4+dq2.*dq3.*t32.*t36.*t38.*6.222952725e-4-dq2.*dq5.*t32.*t33.*t39.*1.2735850275e-3+dq2.*dq4.*t31.*t36.*t39.*6.222952725e-4+dq2.*dq4.*t32.*t36.*t38.*6.222952725e-4+dq2.*dq5.*t32.*t34.*t39.*1.64952e-6+dq2.*dq6.*t31.*t38.*t40.*6.222952725e-4-dq2.*dq6.*t32.*t39.*t40.*6.222952725e-4-t4.*t5.*t6.*t11.*t136.*4.975985e-4+t4.*t5.*t6.*t11.*t137.*4.975985e-4+t4.*t5.*t6.*t11.*t138.*4.975985e-4+t4.*t5.*t8.*t11.*t136.*5.1892415e-3+t4.*t6.*t7.*t11.*t136.*5.1892415e-3-t4.*t5.*t6.*t11.*t139.*4.975985e-4-t4.*t5.*t8.*t11.*t137.*5.1892415e-3-t4.*t6.*t7.*t11.*t137.*5.1892415e-3-t4.*t5.*t8.*t11.*t138.*5.1892415e-3-t4.*t6.*t7.*t11.*t138.*5.1892415e-3+t4.*t7.*t8.*t11.*t136.*4.975985e-4+t4.*t5.*t8.*t11.*t139.*5.1892415e-3+t4.*t6.*t7.*t11.*t139.*5.1892415e-3-t4.*t7.*t8.*t11.*t137.*4.975985e-4-t4.*t7.*t8.*t11.*t138.*4.975985e-4-t5.*t8.*t9.*t10.*t136.*2.384424e-5-t6.*t7.*t9.*t10.*t136.*2.384424e-5+t4.*t7.*t8.*t11.*t139.*4.975985e-4+t5.*t8.*t9.*t10.*t137.*2.384424e-5+t6.*t7.*t9.*t10.*t137.*2.384424e-5+t5.*t8.*t9.*t10.*t138.*2.384424e-5+t6.*t7.*t9.*t10.*t138.*2.384424e-5+t5.*t8.*t9.*t10.*t139.*2.384424e-5+t6.*t7.*t9.*t10.*t139.*2.384424e-5+t4.*t5.*t8.*t40.*t136.*4.14863515e-4+t4.*t6.*t7.*t40.*t136.*4.14863515e-4+t5.*t6.*t11.*t34.*t137.*2.384424e-5-t4.*t5.*t8.*t40.*t137.*4.14863515e-4-t4.*t6.*t7.*t40.*t137.*4.14863515e-4+t5.*t6.*t11.*t34.*t138.*2.384424e-5-t4.*t5.*t8.*t40.*t138.*4.14863515e-4-t4.*t6.*t7.*t40.*t138.*4.14863515e-4-t7.*t8.*t11.*t34.*t137.*2.384424e-5-t7.*t8.*t11.*t34.*t138.*2.384424e-5+t5.*t6.*t33.*t36.*t137.*2.074317575e-4+t5.*t6.*t33.*t36.*t138.*2.074317575e-4-t7.*t8.*t33.*t36.*t137.*2.074317575e-4-t7.*t8.*t33.*t36.*t138.*2.074317575e-4+dq2.*dq5.*t4.*t5.*t6.*t11.*7.10855e-4+dq3.*dq4.*t4.*t5.*t6.*t11.*9.95197e-4-dq3.*dq4.*t4.*t5.*t8.*t11.*1.0378483e-2-dq3.*dq4.*t4.*t6.*t7.*t11.*1.0378483e-2-dq2.*dq5.*t4.*t7.*t8.*t11.*7.10855e-4-dq3.*dq4.*t4.*t7.*t8.*t11.*9.95197e-4+dq2.*dq3.*t5.*t8.*t9.*t11.*7.10855e-4+dq2.*dq3.*t6.*t7.*t9.*t11.*7.10855e-4-dq2.*dq6.*t5.*t6.*t9.*t10.*7.10855e-4+dq2.*dq4.*t5.*t8.*t9.*t11.*7.10855e-4+dq2.*dq4.*t6.*t7.*t9.*t11.*7.10855e-4+dq3.*dq4.*t5.*t8.*t9.*t10.*4.768848e-5+dq3.*dq4.*t6.*t7.*t9.*t10.*4.768848e-5+dq3.*dq6.*t5.*t6.*t9.*t11.*4.768848e-5-dq5.*dq7.*t4.*t5.*t8.*t11.*5.0e-6-dq5.*dq7.*t4.*t6.*t7.*t11.*5.0e-6+dq3.*dq7.*t5.*t6.*t9.*t11.*5.0e-6+dq4.*dq6.*t5.*t6.*t9.*t11.*4.768848e-5+dq5.*dq6.*t5.*t6.*t9.*t10.*9.95197e-4+dq2.*dq6.*t7.*t8.*t9.*t10.*7.10855e-4+dq4.*dq7.*t5.*t6.*t9.*t11.*5.0e-6-dq5.*dq6.*t5.*t8.*t9.*t10.*1.0378483e-2-dq5.*dq6.*t6.*t7.*t9.*t10.*1.0378483e-2-dq3.*dq6.*t7.*t8.*t9.*t11.*4.768848e-5-dq3.*dq7.*t7.*t8.*t9.*t11.*5.0e-6-dq4.*dq6.*t7.*t8.*t9.*t11.*4.768848e-5-dq5.*dq6.*t7.*t8.*t9.*t10.*9.95197e-4+dq6.*dq7.*t5.*t8.*t9.*t10.*5.0e-6+dq6.*dq7.*t6.*t7.*t9.*t10.*5.0e-6-dq4.*dq7.*t7.*t8.*t9.*t11.*5.0e-6+dq2.*dq5.*t4.*t6.*t11.*t31.*4.4783865e-3+dq3.*dq6.*t4.*t5.*t6.*t36.*8.2972703e-4+dq4.*dq6.*t4.*t5.*t6.*t36.*8.2972703e-4-dq2.*dq5.*t4.*t8.*t11.*t32.*4.4783865e-3+dq2.*dq3.*t6.*t9.*t11.*t32.*8.956773e-3+dq3.*dq4.*t5.*t6.*t11.*t34.*4.768848e-5+dq2.*dq3.*t8.*t9.*t11.*t31.*8.956773e-3+dq2.*dq4.*t6.*t9.*t11.*t32.*4.4783865e-3-dq2.*dq6.*t6.*t9.*t10.*t31.*4.4783865e-3-dq3.*dq4.*t4.*t5.*t8.*t40.*8.2972703e-4-dq3.*dq4.*t4.*t6.*t7.*t40.*8.2972703e-4-dq3.*dq6.*t4.*t7.*t8.*t36.*8.2972703e-4+dq2.*dq4.*t8.*t9.*t11.*t31.*4.4783865e-3-dq3.*dq5.*t5.*t8.*t11.*t33.*4.768848e-5-dq3.*dq5.*t6.*t7.*t11.*t33.*4.768848e-5-dq4.*dq6.*t4.*t7.*t8.*t36.*8.2972703e-4+dq3.*dq6.*t5.*t8.*t10.*t34.*2.384424e-5+dq3.*dq6.*t6.*t7.*t10.*t34.*2.384424e-5-dq4.*dq5.*t5.*t8.*t11.*t33.*4.768848e-5-dq4.*dq5.*t6.*t7.*t11.*t33.*4.768848e-5+dq2.*dq6.*t8.*t9.*t10.*t32.*4.4783865e-3-dq3.*dq4.*t7.*t8.*t11.*t34.*4.768848e-5+dq4.*dq6.*t5.*t8.*t10.*t34.*2.384424e-5+dq4.*dq6.*t6.*t7.*t10.*t34.*2.384424e-5-dq5.*dq6.*t5.*t8.*t9.*t36.*8.2972703e-4-dq5.*dq6.*t6.*t7.*t9.*t36.*8.2972703e-4+dq3.*dq4.*t5.*t6.*t33.*t36.*4.14863515e-4+dq2.*dq3.*t4.*t10.*t31.*t38.*4.768848e-5+dq2.*dq4.*t4.*t10.*t31.*t38.*4.768848e-5-dq2.*dq3.*t4.*t10.*t32.*t39.*4.768848e-5-dq2.*dq4.*t4.*t10.*t32.*t39.*4.768848e-5+dq2.*dq5.*t4.*t11.*t31.*t38.*4.975985e-4-dq3.*dq4.*t7.*t8.*t33.*t36.*4.14863515e-4+dq3.*dq5.*t5.*t8.*t34.*t36.*4.14863515e-4+dq3.*dq5.*t6.*t7.*t34.*t36.*4.14863515e-4-dq2.*dq5.*t4.*t11.*t31.*t39.*5.1892415e-3-dq2.*dq5.*t4.*t11.*t32.*t38.*5.1892415e-3+dq4.*dq5.*t5.*t8.*t34.*t36.*4.14863515e-4+dq4.*dq5.*t6.*t7.*t34.*t36.*4.14863515e-4-dq2.*dq5.*t4.*t11.*t32.*t39.*4.975985e-4-dq2.*dq6.*t4.*t11.*t31.*t39.*2.384424e-5-dq2.*dq6.*t4.*t11.*t32.*t38.*2.384424e-5+dq2.*dq3.*t9.*t11.*t31.*t38.*1.0378483e-2+dq2.*dq3.*t9.*t11.*t31.*t39.*9.95197e-4+dq2.*dq3.*t9.*t11.*t32.*t38.*9.95197e-4+dq2.*dq4.*t9.*t11.*t31.*t38.*1.0378483e-2-dq3.*dq6.*t5.*t8.*t33.*t40.*4.14863515e-4-dq3.*dq6.*t6.*t7.*t33.*t40.*4.14863515e-4-dq2.*dq3.*t9.*t11.*t32.*t39.*1.0378483e-2+dq2.*dq4.*t9.*t11.*t31.*t39.*9.95197e-4+dq2.*dq4.*t9.*t11.*t32.*t38.*9.95197e-4+dq2.*dq5.*t9.*t10.*t31.*t39.*2.384424e-5+dq2.*dq5.*t9.*t10.*t32.*t38.*2.384424e-5-dq2.*dq6.*t9.*t10.*t31.*t38.*4.975985e-4-dq4.*dq6.*t5.*t8.*t33.*t40.*4.14863515e-4-dq4.*dq6.*t6.*t7.*t33.*t40.*4.14863515e-4-dq2.*dq4.*t9.*t11.*t32.*t39.*1.0378483e-2+dq2.*dq6.*t9.*t10.*t31.*t39.*5.1892415e-3+dq2.*dq6.*t9.*t10.*t32.*t38.*5.1892415e-3+dq2.*dq6.*t9.*t10.*t32.*t39.*4.975985e-4-dq2.*dq3.*t11.*t31.*t33.*t39.*2.384424e-5-dq2.*dq3.*t11.*t32.*t33.*t38.*2.384424e-5-dq2.*dq4.*t11.*t31.*t33.*t39.*2.384424e-5-dq2.*dq4.*t11.*t32.*t33.*t38.*2.384424e-5+dq2.*dq6.*t10.*t31.*t33.*t38.*1.192212e-5-dq2.*dq5.*t4.*t31.*t39.*t40.*4.14863515e-4-dq2.*dq5.*t4.*t32.*t38.*t40.*4.14863515e-4+dq2.*dq5.*t11.*t31.*t34.*t38.*2.384424e-5-dq2.*dq6.*t10.*t32.*t33.*t39.*1.192212e-5+dq2.*dq3.*t9.*t31.*t38.*t40.*8.2972703e-4-dq2.*dq5.*t11.*t32.*t34.*t39.*2.384424e-5+dq2.*dq6.*t9.*t31.*t36.*t39.*8.2972703e-4+dq2.*dq6.*t9.*t32.*t36.*t38.*8.2972703e-4+dq2.*dq4.*t9.*t31.*t38.*t40.*8.2972703e-4-dq2.*dq3.*t9.*t32.*t39.*t40.*8.2972703e-4-dq2.*dq4.*t9.*t32.*t39.*t40.*8.2972703e-4+dq2.*dq3.*t31.*t34.*t36.*t39.*2.074317575e-4+dq2.*dq3.*t32.*t34.*t36.*t38.*2.074317575e-4+dq2.*dq5.*t31.*t33.*t36.*t38.*2.074317575e-4+dq2.*dq4.*t31.*t34.*t36.*t39.*2.074317575e-4+dq2.*dq4.*t32.*t34.*t36.*t38.*2.074317575e-4-dq2.*dq5.*t32.*t33.*t36.*t39.*2.074317575e-4+dq2.*dq6.*t31.*t34.*t38.*t40.*2.074317575e-4-dq2.*dq6.*t32.*t34.*t39.*t40.*2.074317575e-4;t140+t141+t142+t143+t144+t145+t146+t147+t148+t149+t150+t151+t152+t153+t154+t155+t156+t157+t158+t159+t160+t161+t162+t163+t164+t165+t166+t167+t168+t169+t170+t171+t172+t173+t174+t175+t176+t177+t178+t179+t180+t181+t182+t183+t184+t185+t186+t187+t188+t189+t190+t191+t192+t193+t194+t195+t196+t197-t4.*t136.*4.62678618e-3-t5.*t135.*1.6296175e-3+t7.*t135.*1.20304975e-1-t6.*t138.*4.46189562e-1-t8.*t138.*7.476336e-2-t10.*t139.*4.975985e-4-t31.*t135.*1.00391957e-2+t32.*t135.*7.03321055045e-1-dq3.*dq5.*t4.*3.2074e-5-dq3.*dq4.*t6.*8.92379124e-1-dq4.*dq5.*t4.*3.2074e-5-dq3.*dq4.*t8.*1.4952672e-1-dq5.*dq6.*t4.*1.23472703e-3-dq3.*dq5.*t9.*1.254015e-3-dq4.*dq5.*t9.*1.254015e-3-dq3.*dq6.*t11.*1.0378483e-2-dq4.*dq6.*t11.*1.0378483e-2-dq3.*dq5.*t34.*3.29904e-6-dq4.*dq5.*t34.*3.29904e-6-dq3.*dq6.*t40.*4.14863515e-4-dq4.*dq6.*t40.*4.14863515e-4+t4.*t8.*t136.*5.6430675e-3+t4.*t8.*t138.*5.6430675e-3-t4.*t10.*t136.*2.384424e-5-t7.*t8.*t135.*3.541187e-2-t8.*t9.*t136.*1.44333e-4-t6.*t10.*t138.*4.4783865e-3-t6.*t10.*t139.*4.4783865e-3-t8.*t9.*t138.*1.44333e-4-t9.*t11.*t136.*5.1892415e-3-t9.*t11.*t139.*5.1892415e-3+t6.*t31.*t135.*4.46189562e-1+t6.*t32.*t135.*7.476336e-2+t8.*t31.*t135.*7.476336e-2-t8.*t32.*t135.*4.46189562e-1-t9.*t40.*t136.*4.14863515e-4-t31.*t39.*t135.*1.8083421453625e-1-t32.*t38.*t135.*1.8083421453625e-1-t32.*t39.*t135.*4.99715694e-2+dq2.*dq5.*t4.*t7.*1.1286135e-2-dq3.*dq5.*t4.*t6.*2.88666e-4+dq3.*dq4.*t4.*t8.*1.1286135e-2-dq4.*dq5.*t4.*t6.*2.88666e-4-dq2.*dq5.*t5.*t8.*1.0581988725e-2-dq2.*dq5.*t6.*t7.*1.0581988725e-2-dq2.*dq5.*t7.*t9.*2.88666e-4-dq3.*dq4.*t6.*t10.*8.956773e-3-dq3.*dq5.*t6.*t9.*1.1286135e-2-dq3.*dq4.*t8.*t9.*2.88666e-4-dq4.*dq5.*t6.*t9.*1.1286135e-2-dq5.*dq6.*t4.*t10.*1.0378483e-2+dq3.*dq6.*t8.*t11.*8.956773e-3-dq3.*dq6.*t9.*t10.*9.95197e-4+dq4.*dq6.*t8.*t11.*8.956773e-3-dq4.*dq6.*t9.*t10.*9.95197e-4-dq5.*dq6.*t4.*t36.*8.2972703e-4-t4.*t5.*t8.*t135.*4.478625e-4-t4.*t6.*t7.*t135.*4.478625e-4-t7.*t8.*t10.*t135.*3.554275e-4+t8.*t9.*t11.*t136.*4.4783865e-3+t8.*t9.*t11.*t138.*4.4783865e-3+t8.*t9.*t11.*t139.*4.4783865e-3-t4.*t6.*t32.*t135.*5.6430675e-3-t4.*t8.*t31.*t135.*5.6430675e-3+t6.*t9.*t32.*t135.*1.44333e-4+t6.*t10.*t31.*t135.*4.4783865e-3+t8.*t9.*t31.*t135.*1.44333e-4-t8.*t10.*t32.*t135.*4.4783865e-3-t4.*t31.*t38.*t135.*4.62678618e-3-t4.*t31.*t39.*t135.*6.270075e-4-t4.*t32.*t38.*t135.*6.270075e-4-t9.*t32.*t39.*t135.*1.0579838e-4-t10.*t31.*t39.*t135.*5.1892415e-3-t10.*t32.*t38.*t135.*5.1892415e-3-t10.*t32.*t39.*t135.*4.975985e-4-t31.*t33.*t39.*t135.*8.2476e-7-t32.*t33.*t38.*t135.*8.2476e-7-t31.*t34.*t39.*t135.*6.3679251375e-4-t32.*t34.*t38.*t135.*6.3679251375e-4-t31.*t36.*t39.*t135.*3.1114763625e-4-t32.*t36.*t38.*t135.*3.1114763625e-4-dq2.*dq5.*t4.*t7.*t8.*9.25357236e-3-dq2.*dq5.*t5.*t6.*t9.*2.1159676e-4-dq2.*dq6.*t4.*t7.*t8.*1.23472703e-3-dq2.*dq5.*t5.*t8.*t9.*3.2074e-5-dq2.*dq5.*t6.*t7.*t9.*3.2074e-5+dq2.*dq6.*t4.*t7.*t10.*8.956773e-3+dq3.*dq5.*t4.*t6.*t11.*8.956773e-3+dq4.*dq5.*t4.*t6.*t11.*8.956773e-3-dq2.*dq6.*t5.*t8.*t10.*2.384424e-5-dq2.*dq6.*t6.*t7.*t10.*2.384424e-5-dq2.*dq7.*t5.*t8.*t10.*5.0e-6-dq2.*dq7.*t6.*t7.*t10.*5.0e-6+dq5.*dq6.*t4.*t8.*t10.*8.956773e-3+dq2.*dq5.*t7.*t9.*t11.*8.956773e-3-dq3.*dq6.*t6.*t9.*t10.*8.956773e-3+dq3.*dq4.*t8.*t9.*t11.*8.956773e-3-dq4.*dq6.*t6.*t9.*t10.*8.956773e-3-t5.*t8.*t9.*t11.*t135.*3.554275e-4-t6.*t7.*t9.*t11.*t135.*3.554275e-4-t6.*t9.*t11.*t32.*t135.*4.4783865e-3-t8.*t9.*t11.*t31.*t135.*4.4783865e-3-t4.*t10.*t31.*t38.*t135.*2.384424e-5-t9.*t11.*t31.*t38.*t135.*5.1892415e-3-t9.*t11.*t31.*t39.*t135.*4.975985e-4-t9.*t11.*t32.*t38.*t135.*4.975985e-4-t9.*t31.*t38.*t40.*t135.*4.14863515e-4-t31.*t34.*t36.*t39.*t135.*1.0371587875e-4-t32.*t34.*t36.*t38.*t135.*1.0371587875e-4-dq2.*dq5.*t4.*t7.*t8.*t10.*4.768848e-5-dq2.*dq6.*t4.*t7.*t8.*t10.*1.0378483e-2-dq2.*dq7.*t5.*t6.*t9.*t11.*5.0e-6-dq2.*dq5.*t7.*t8.*t9.*t11.*1.0378483e-2-dq2.*dq6.*t4.*t7.*t8.*t36.*8.2972703e-4-dq2.*dq5.*t5.*t8.*t11.*t33.*4.768848e-5-dq2.*dq5.*t6.*t7.*t11.*t33.*4.768848e-5-dq2.*dq5.*t7.*t8.*t9.*t40.*8.2972703e-4-dq2.*dq6.*t5.*t8.*t33.*t40.*4.14863515e-4-dq2.*dq6.*t6.*t7.*t33.*t40.*4.14863515e-4;t140+t141+t142+t143+t144+t145+t146+t147+t148+t149+t150+t151+t152+t153+t154+t155+t156+t157+t158+t159+t160+t161+t162+t163+t164+t165+t166+t167+t168+t169+t170+t171+t172+t173+t174+t175+t176+t177+t178+t179+t180+t181+t182+t183+t184+t185+t186+t187+t188+t189+t190+t191+t192+t193+t194+t195+t196+t197-t4.*t136.*4.62678618e-3+t6.*t135.*2.23094781e-1+t6.*t137.*4.46189562e-1+t8.*t135.*3.738168e-2+t8.*t137.*7.476336e-2-t10.*t139.*4.975985e-4-dq3.*dq5.*t4.*3.2074e-5-dq4.*dq5.*t4.*3.2074e-5-dq5.*dq6.*t4.*1.23472703e-3-dq3.*dq5.*t9.*1.254015e-3-dq4.*dq5.*t9.*1.254015e-3-dq3.*dq6.*t11.*1.0378483e-2-dq4.*dq6.*t11.*1.0378483e-2-dq3.*dq5.*t34.*3.29904e-6-dq4.*dq5.*t34.*3.29904e-6-dq3.*dq6.*t40.*4.14863515e-4-dq4.*dq6.*t40.*4.14863515e-4-t4.*t8.*t135.*2.82153375e-3-t4.*t8.*t137.*5.6430675e-3-t4.*t10.*t136.*2.384424e-5-t7.*t8.*t135.*3.541187e-2+t6.*t10.*t135.*2.23919325e-3+t8.*t9.*t135.*7.21665e-5+t6.*t10.*t137.*4.4783865e-3+t8.*t9.*t137.*1.44333e-4-t9.*t11.*t136.*5.1892415e-3-t9.*t11.*t139.*5.1892415e-3+t6.*t31.*t135.*2.23094781e-1+t6.*t32.*t135.*3.738168e-2+t8.*t31.*t135.*3.738168e-2-t8.*t32.*t135.*2.23094781e-1-t9.*t40.*t136.*4.14863515e-4-t31.*t39.*t135.*1.8083421453625e-1-t32.*t38.*t135.*1.8083421453625e-1-t32.*t39.*t135.*4.99715694e-2-dq2.*dq5.*t5.*t8.*1.0581988725e-2-dq2.*dq5.*t6.*t7.*1.0581988725e-2-dq5.*dq6.*t4.*t10.*1.0378483e-2-dq3.*dq6.*t9.*t10.*9.95197e-4-dq4.*dq6.*t9.*t10.*9.95197e-4-dq5.*dq6.*t4.*t36.*8.2972703e-4-t4.*t5.*t8.*t135.*4.478625e-4-t4.*t6.*t7.*t135.*4.478625e-4-t7.*t8.*t10.*t135.*3.554275e-4-t8.*t9.*t11.*t135.*2.23919325e-3-t8.*t9.*t11.*t137.*4.4783865e-3-t4.*t6.*t32.*t135.*2.82153375e-3-t4.*t8.*t31.*t135.*2.82153375e-3+t6.*t9.*t32.*t135.*7.21665e-5+t6.*t10.*t31.*t135.*2.23919325e-3+t8.*t9.*t31.*t135.*7.21665e-5-t8.*t10.*t32.*t135.*2.23919325e-3-t4.*t31.*t38.*t135.*4.62678618e-3-t4.*t31.*t39.*t135.*6.270075e-4-t4.*t32.*t38.*t135.*6.270075e-4-t9.*t32.*t39.*t135.*1.0579838e-4-t10.*t31.*t39.*t135.*5.1892415e-3-t10.*t32.*t38.*t135.*5.1892415e-3-t10.*t32.*t39.*t135.*4.975985e-4-t31.*t33.*t39.*t135.*8.2476e-7-t32.*t33.*t38.*t135.*8.2476e-7-t31.*t34.*t39.*t135.*6.3679251375e-4-t32.*t34.*t38.*t135.*6.3679251375e-4-t31.*t36.*t39.*t135.*3.1114763625e-4-t32.*t36.*t38.*t135.*3.1114763625e-4-dq2.*dq5.*t4.*t7.*t8.*9.25357236e-3-dq2.*dq5.*t5.*t6.*t9.*2.1159676e-4-dq2.*dq6.*t4.*t7.*t8.*1.23472703e-3-dq2.*dq5.*t5.*t8.*t9.*3.2074e-5-dq2.*dq5.*t6.*t7.*t9.*3.2074e-5-dq2.*dq6.*t5.*t8.*t10.*2.384424e-5-dq2.*dq6.*t6.*t7.*t10.*2.384424e-5-dq2.*dq7.*t5.*t8.*t10.*5.0e-6-dq2.*dq7.*t6.*t7.*t10.*5.0e-6-t5.*t8.*t9.*t11.*t135.*3.554275e-4-t6.*t7.*t9.*t11.*t135.*3.554275e-4-t6.*t9.*t11.*t32.*t135.*2.23919325e-3-t8.*t9.*t11.*t31.*t135.*2.23919325e-3-t4.*t10.*t31.*t38.*t135.*2.384424e-5-t9.*t11.*t31.*t38.*t135.*5.1892415e-3-t9.*t11.*t31.*t39.*t135.*4.975985e-4-t9.*t11.*t32.*t38.*t135.*4.975985e-4-t9.*t31.*t38.*t40.*t135.*4.14863515e-4-t31.*t34.*t36.*t39.*t135.*1.0371587875e-4-t32.*t34.*t36.*t38.*t135.*1.0371587875e-4-dq2.*dq5.*t4.*t7.*t8.*t10.*4.768848e-5-dq2.*dq6.*t4.*t7.*t8.*t10.*1.0378483e-2-dq2.*dq7.*t5.*t6.*t9.*t11.*5.0e-6-dq2.*dq5.*t7.*t8.*t9.*t11.*1.0378483e-2-dq2.*dq6.*t4.*t7.*t8.*t36.*8.2972703e-4-dq2.*dq5.*t5.*t8.*t11.*t33.*4.768848e-5-dq2.*dq5.*t6.*t7.*t11.*t33.*4.768848e-5-dq2.*dq5.*t7.*t8.*t9.*t40.*8.2972703e-4-dq2.*dq6.*t5.*t8.*t33.*t40.*4.14863515e-4-dq2.*dq6.*t6.*t7.*t33.*t40.*4.14863515e-4;t4.*t135.*8.0185e-6+t4.*t137.*1.6037e-5+t4.*t138.*1.6037e-5+t9.*t135.*3.1350375e-4+t9.*t137.*6.270075e-4+t9.*t138.*6.270075e-4-t11.*t139.*2.384424e-5+t33.*t135.*6.3679251375e-4-t34.*t135.*8.2476e-7-t33.*t137.*1.2735850275e-3-t33.*t138.*1.2735850275e-3+t34.*t137.*1.64952e-6+t34.*t138.*1.64952e-6+dq3.*dq4.*t4.*3.2074e-5+dq3.*dq6.*t4.*1.23472703e-3+dq4.*dq6.*t4.*1.23472703e-3+dq3.*dq4.*t9.*1.254015e-3-dq6.*dq7.*t11.*5.0e-6-dq3.*dq4.*t33.*2.547170055e-3+dq3.*dq4.*t34.*3.29904e-6+dq5.*dq6.*t40.*8.2972703e-4+t4.*t6.*t135.*7.21665e-5+t4.*t6.*t137.*1.44333e-4-t4.*t11.*t135.*2.4879925e-4+t6.*t9.*t135.*2.82153375e-3-t4.*t11.*t137.*4.975985e-4+t6.*t9.*t137.*5.6430675e-3-t4.*t11.*t138.*4.975985e-4+t11.*t34.*t135.*1.192212e-5-t11.*t34.*t137.*2.384424e-5-t11.*t34.*t138.*2.384424e-5+t33.*t36.*t135.*1.0371587875e-4-t33.*t36.*t137.*2.074317575e-4-t33.*t36.*t138.*2.074317575e-4-dq2.*dq3.*t4.*t7.*1.1286135e-2+dq2.*dq3.*t5.*t8.*1.0581988725e-2+dq2.*dq3.*t6.*t7.*1.0581988725e-2+dq2.*dq4.*t5.*t8.*1.0581988725e-2+dq2.*dq4.*t6.*t7.*1.0581988725e-2+dq2.*dq3.*t7.*t9.*2.88666e-4-dq3.*dq4.*t4.*t11.*9.95197e-4-dq3.*dq6.*t9.*t11.*4.768848e-5-dq3.*dq7.*t9.*t11.*5.0e-6-dq4.*dq6.*t9.*t11.*4.768848e-5-dq4.*dq7.*t9.*t11.*5.0e-6-dq3.*dq6.*t4.*t36.*8.2972703e-4-dq4.*dq6.*t4.*t36.*8.2972703e-4-dq3.*dq4.*t11.*t34.*4.768848e-5-dq3.*dq4.*t33.*t36.*4.14863515e-4+t4.*t5.*t6.*t135.*1.1455e-5-t4.*t7.*t8.*t135.*1.1455e-5+t5.*t6.*t9.*t135.*4.478625e-4-t4.*t6.*t11.*t135.*2.23919325e-3-t4.*t6.*t11.*t137.*4.4783865e-3-t7.*t8.*t9.*t135.*4.478625e-4+t4.*t6.*t31.*t135.*7.21665e-5-t4.*t8.*t32.*t135.*7.21665e-5+t6.*t9.*t31.*t135.*2.82153375e-3-t8.*t9.*t32.*t135.*2.82153375e-3+t4.*t31.*t38.*t135.*8.0185e-6-t4.*t31.*t39.*t135.*5.289919e-5-t4.*t32.*t38.*t135.*5.289919e-5-t4.*t32.*t39.*t135.*8.0185e-6+t9.*t31.*t38.*t135.*3.1350375e-4-t9.*t31.*t39.*t135.*2.31339309e-3-t9.*t32.*t38.*t135.*2.31339309e-3-t9.*t32.*t39.*t135.*3.1350375e-4-t31.*t33.*t38.*t135.*6.3679251375e-4+t31.*t34.*t38.*t135.*8.2476e-7+t32.*t33.*t39.*t135.*6.3679251375e-4-t32.*t34.*t39.*t135.*8.2476e-7-dq2.*dq3.*t4.*t5.*t6.*9.25357236e-3-dq2.*dq4.*t4.*t5.*t6.*9.25357236e-3-dq2.*dq3.*t4.*t5.*t8.*1.254015e-3-dq2.*dq3.*t4.*t6.*t7.*1.254015e-3-dq2.*dq4.*t4.*t5.*t8.*1.254015e-3-dq2.*dq4.*t4.*t6.*t7.*1.254015e-3+dq2.*dq3.*t4.*t7.*t8.*9.25357236e-3+dq2.*dq3.*t5.*t6.*t9.*2.1159676e-4+dq2.*dq4.*t4.*t7.*t8.*9.25357236e-3+dq2.*dq4.*t5.*t6.*t9.*2.1159676e-4+dq2.*dq3.*t5.*t8.*t9.*3.2074e-5+dq2.*dq3.*t6.*t7.*t9.*3.2074e-5+dq2.*dq4.*t5.*t8.*t9.*3.2074e-5+dq2.*dq4.*t6.*t7.*t9.*3.2074e-5-dq2.*dq3.*t7.*t8.*t9.*2.1159676e-4-dq2.*dq4.*t7.*t8.*t9.*2.1159676e-4+dq2.*dq6.*t5.*t8.*t9.*1.23472703e-3+dq2.*dq6.*t6.*t7.*t9.*1.23472703e-3-dq2.*dq3.*t7.*t9.*t11.*8.956773e-3-dq2.*dq3.*t5.*t8.*t33.*3.29904e-6-dq2.*dq3.*t6.*t7.*t33.*3.29904e-6-dq2.*dq3.*t5.*t8.*t34.*2.547170055e-3-dq2.*dq3.*t6.*t7.*t34.*2.547170055e-3-dq2.*dq4.*t5.*t8.*t33.*3.29904e-6-dq2.*dq4.*t6.*t7.*t33.*3.29904e-6-dq2.*dq4.*t5.*t8.*t34.*2.547170055e-3-dq2.*dq4.*t6.*t7.*t34.*2.547170055e-3-dq2.*dq3.*t5.*t8.*t36.*4.14863515e-4-dq2.*dq3.*t6.*t7.*t36.*4.14863515e-4-dq2.*dq4.*t5.*t8.*t36.*4.14863515e-4-dq2.*dq4.*t6.*t7.*t36.*4.14863515e-4-dq2.*dq6.*t5.*t6.*t40.*8.2972703e-4+dq2.*dq6.*t7.*t8.*t40.*8.2972703e-4-t4.*t5.*t6.*t11.*t135.*3.554275e-4+t4.*t7.*t8.*t11.*t135.*3.554275e-4-t4.*t6.*t11.*t31.*t135.*2.23919325e-3+t4.*t8.*t11.*t32.*t135.*2.23919325e-3-t4.*t11.*t31.*t38.*t135.*2.4879925e-4+t4.*t11.*t31.*t39.*t135.*2.59462075e-3+t4.*t11.*t32.*t38.*t135.*2.59462075e-3+t4.*t11.*t32.*t39.*t135.*2.4879925e-4-t9.*t10.*t31.*t39.*t135.*1.192212e-5-t9.*t10.*t32.*t38.*t135.*1.192212e-5+t4.*t31.*t39.*t40.*t135.*2.074317575e-4+t4.*t32.*t38.*t40.*t135.*2.074317575e-4-t11.*t31.*t34.*t38.*t135.*1.192212e-5+t11.*t32.*t34.*t39.*t135.*1.192212e-5-t31.*t33.*t36.*t38.*t135.*1.0371587875e-4+t32.*t33.*t36.*t39.*t135.*1.0371587875e-4-dq2.*dq3.*t4.*t5.*t6.*t10.*4.768848e-5-dq2.*dq4.*t4.*t5.*t6.*t10.*4.768848e-5+dq2.*dq3.*t4.*t7.*t8.*t10.*4.768848e-5+dq2.*dq4.*t4.*t7.*t8.*t10.*4.768848e-5-dq2.*dq3.*t5.*t6.*t9.*t11.*1.0378483e-2+dq2.*dq6.*t4.*t5.*t8.*t11.*4.768848e-5+dq2.*dq6.*t4.*t6.*t7.*t11.*4.768848e-5-dq2.*dq4.*t5.*t6.*t9.*t11.*1.0378483e-2+dq2.*dq7.*t4.*t5.*t8.*t11.*5.0e-6+dq2.*dq7.*t4.*t6.*t7.*t11.*5.0e-6-dq2.*dq3.*t5.*t8.*t9.*t11.*9.95197e-4-dq2.*dq3.*t6.*t7.*t9.*t11.*9.95197e-4-dq2.*dq4.*t5.*t8.*t9.*t11.*9.95197e-4-dq2.*dq4.*t6.*t7.*t9.*t11.*9.95197e-4+dq2.*dq3.*t7.*t8.*t9.*t11.*1.0378483e-2+dq2.*dq4.*t7.*t8.*t9.*t11.*1.0378483e-2+dq2.*dq3.*t5.*t8.*t11.*t33.*4.768848e-5+dq2.*dq3.*t6.*t7.*t11.*t33.*4.768848e-5+dq2.*dq4.*t5.*t8.*t11.*t33.*4.768848e-5+dq2.*dq4.*t6.*t7.*t11.*t33.*4.768848e-5-dq2.*dq3.*t5.*t6.*t9.*t40.*8.2972703e-4-dq2.*dq4.*t5.*t6.*t9.*t40.*8.2972703e-4-dq2.*dq6.*t5.*t8.*t9.*t36.*8.2972703e-4-dq2.*dq6.*t6.*t7.*t9.*t36.*8.2972703e-4+dq2.*dq3.*t7.*t8.*t9.*t40.*8.2972703e-4+dq2.*dq4.*t7.*t8.*t9.*t40.*8.2972703e-4-dq2.*dq3.*t5.*t8.*t34.*t36.*4.14863515e-4-dq2.*dq3.*t6.*t7.*t34.*t36.*4.14863515e-4-dq2.*dq4.*t5.*t8.*t34.*t36.*4.14863515e-4-dq2.*dq4.*t6.*t7.*t34.*t36.*4.14863515e-4;t11.*t135.*2.59462075e-3+t11.*t137.*5.1892415e-3+t11.*t138.*5.1892415e-3-t40.*t135.*1.0371587875e-4-t40.*t136.*4.14863515e-4+t40.*t137.*2.074317575e-4+t40.*t138.*2.074317575e-4-dq3.*dq5.*t4.*1.23472703e-3-dq4.*dq5.*t4.*1.23472703e-3+dq3.*dq4.*t11.*1.0378483e-2+dq5.*dq7.*t11.*5.0e-6+dq3.*dq4.*t40.*4.14863515e-4-t8.*t11.*t135.*2.23919325e-3+t9.*t10.*t135.*2.4879925e-4-t8.*t11.*t137.*4.4783865e-3+t9.*t10.*t137.*4.975985e-4+t9.*t10.*t138.*4.975985e-4+t10.*t33.*t135.*5.96106e-6-t10.*t33.*t137.*1.192212e-5-t10.*t33.*t138.*1.192212e-5+t34.*t40.*t135.*1.0371587875e-4-t34.*t40.*t137.*2.074317575e-4-t34.*t40.*t138.*2.074317575e-4-dq3.*dq7.*t4.*t10.*5.0e-6-dq4.*dq7.*t4.*t10.*5.0e-6+dq3.*dq4.*t9.*t10.*9.95197e-4+dq3.*dq5.*t9.*t11.*4.768848e-5+dq4.*dq5.*t9.*t11.*4.768848e-5+dq3.*dq5.*t4.*t36.*8.2972703e-4+dq4.*dq5.*t4.*t36.*8.2972703e-4-dq3.*dq4.*t10.*t33.*2.384424e-5-dq3.*dq4.*t34.*t40.*4.14863515e-4-t5.*t8.*t11.*t135.*3.554275e-4-t6.*t7.*t11.*t135.*3.554275e-4+t6.*t9.*t10.*t135.*2.23919325e-3+t6.*t9.*t10.*t137.*4.4783865e-3-t6.*t11.*t32.*t135.*2.23919325e-3-t8.*t11.*t31.*t135.*2.23919325e-3-t11.*t31.*t38.*t135.*2.59462075e-3-t11.*t31.*t39.*t135.*2.4879925e-4-t11.*t32.*t38.*t135.*2.4879925e-4+t11.*t32.*t39.*t135.*2.59462075e-3-t31.*t38.*t40.*t135.*3.1114763625e-4+t32.*t39.*t40.*t135.*3.1114763625e-4-dq2.*dq3.*t4.*t5.*t6.*1.23472703e-3-dq2.*dq4.*t4.*t5.*t6.*1.23472703e-3+dq2.*dq3.*t4.*t7.*t8.*1.23472703e-3+dq2.*dq4.*t4.*t7.*t8.*1.23472703e-3-dq2.*dq3.*t4.*t7.*t10.*8.956773e-3+dq2.*dq3.*t5.*t8.*t10.*2.384424e-5+dq2.*dq3.*t6.*t7.*t10.*2.384424e-5+dq2.*dq4.*t5.*t8.*t10.*2.384424e-5+dq2.*dq4.*t6.*t7.*t10.*2.384424e-5-dq2.*dq5.*t5.*t8.*t9.*1.23472703e-3-dq2.*dq5.*t6.*t7.*t9.*1.23472703e-3-dq2.*dq7.*t5.*t6.*t11.*5.0e-6+dq2.*dq7.*t7.*t8.*t11.*5.0e-6+dq2.*dq5.*t5.*t6.*t40.*8.2972703e-4-dq2.*dq5.*t7.*t8.*t40.*8.2972703e-4+t5.*t6.*t9.*t10.*t135.*3.554275e-4-t7.*t8.*t9.*t10.*t135.*3.554275e-4+t6.*t9.*t10.*t31.*t135.*2.23919325e-3-t8.*t9.*t10.*t32.*t135.*2.23919325e-3+t4.*t11.*t31.*t39.*t135.*1.192212e-5+t4.*t11.*t32.*t38.*t135.*1.192212e-5+t9.*t10.*t31.*t38.*t135.*2.4879925e-4-t9.*t10.*t31.*t39.*t135.*2.59462075e-3-t9.*t10.*t32.*t38.*t135.*2.59462075e-3-t9.*t10.*t32.*t39.*t135.*2.4879925e-4-t10.*t31.*t33.*t38.*t135.*5.96106e-6+t10.*t32.*t33.*t39.*t135.*5.96106e-6-t9.*t31.*t36.*t39.*t135.*4.14863515e-4-t9.*t32.*t36.*t38.*t135.*4.14863515e-4-t31.*t34.*t38.*t40.*t135.*1.0371587875e-4+t32.*t34.*t39.*t40.*t135.*1.0371587875e-4-dq2.*dq3.*t4.*t5.*t6.*t10.*1.0378483e-2-dq2.*dq4.*t4.*t5.*t6.*t10.*1.0378483e-2-dq2.*dq3.*t4.*t5.*t8.*t10.*9.95197e-4-dq2.*dq3.*t4.*t6.*t7.*t10.*9.95197e-4-dq2.*dq4.*t4.*t5.*t8.*t10.*9.95197e-4-dq2.*dq4.*t4.*t6.*t7.*t10.*9.95197e-4+dq2.*dq3.*t4.*t7.*t8.*t10.*1.0378483e-2+dq2.*dq4.*t4.*t7.*t8.*t10.*1.0378483e-2-dq2.*dq5.*t4.*t5.*t8.*t11.*4.768848e-5-dq2.*dq5.*t4.*t6.*t7.*t11.*4.768848e-5-dq2.*dq7.*t5.*t8.*t9.*t10.*5.0e-6-dq2.*dq7.*t6.*t7.*t9.*t10.*5.0e-6-dq2.*dq3.*t4.*t5.*t6.*t36.*8.2972703e-4-dq2.*dq4.*t4.*t5.*t6.*t36.*8.2972703e-4+dq2.*dq3.*t4.*t7.*t8.*t36.*8.2972703e-4+dq2.*dq4.*t4.*t7.*t8.*t36.*8.2972703e-4-dq2.*dq3.*t5.*t8.*t10.*t34.*2.384424e-5-dq2.*dq3.*t6.*t7.*t10.*t34.*2.384424e-5-dq2.*dq4.*t5.*t8.*t10.*t34.*2.384424e-5-dq2.*dq4.*t6.*t7.*t10.*t34.*2.384424e-5+dq2.*dq5.*t5.*t8.*t9.*t36.*8.2972703e-4+dq2.*dq5.*t6.*t7.*t9.*t36.*8.2972703e-4+dq2.*dq3.*t5.*t8.*t33.*t40.*4.14863515e-4+dq2.*dq3.*t6.*t7.*t33.*t40.*4.14863515e-4+dq2.*dq4.*t5.*t8.*t33.*t40.*4.14863515e-4+dq2.*dq4.*t6.*t7.*t33.*t40.*4.14863515e-4;dq5.*dq6.*t11.*(-5.0e-6)+dq3.*dq6.*t4.*t10.*5.0e-6+dq4.*dq6.*t4.*t10.*5.0e-6+dq3.*dq5.*t9.*t11.*5.0e-6+dq4.*dq5.*t9.*t11.*5.0e-6+dq2.*dq3.*t5.*t8.*t10.*5.0e-6+dq2.*dq3.*t6.*t7.*t10.*5.0e-6+dq2.*dq4.*t5.*t8.*t10.*5.0e-6+dq2.*dq4.*t6.*t7.*t10.*5.0e-6+dq2.*dq6.*t5.*t6.*t11.*5.0e-6-dq2.*dq6.*t7.*t8.*t11.*5.0e-6-dq2.*dq5.*t4.*t5.*t8.*t11.*5.0e-6-dq2.*dq5.*t4.*t6.*t7.*t11.*5.0e-6+dq2.*dq3.*t5.*t6.*t9.*t11.*5.0e-6+dq2.*dq4.*t5.*t6.*t9.*t11.*5.0e-6-dq2.*dq3.*t7.*t8.*t9.*t11.*5.0e-6+dq2.*dq6.*t5.*t8.*t9.*t10.*5.0e-6+dq2.*dq6.*t6.*t7.*t9.*t10.*5.0e-6-dq2.*dq4.*t7.*t8.*t9.*t11.*5.0e-6];
end
if nargout > 3
    t198 = dq3.*t9;
    t199 = dq4.*t9;
    t201 = dq2.*t4.*t130;
    t200 = t198+t199-t201;
    t202 = dq3+dq4;
    t203 = dq2.*t131;
    t204 = dq5+t203;
    t205 = dq3.*(2.1e1./1.0e3);
    t206 = dq4.*(2.1e1./1.0e3);
    t207 = t205+t206;
    t208 = dq3.*t4;
    t209 = dq4.*t4;
    t210 = dq2.*t9.*t130;
    t211 = t208+t209+t210;
    t212 = t11.*t211;
    t213 = dq5-t203;
    t214 = t10.*t213;
    t215 = t212+t214;
    t216 = dq2.*dq5.*t4.*t130.*(2.1e1./1.0e3);
    t217 = dq2.*t5.*t8.*t202.*(2.1e1./1.0e3);
    t218 = dq2.*t6.*t7.*t202.*(2.1e1./1.0e3);
    Phim = [0.0;0.0;0.0;dq2.*dq5.*t8.*t131.*(-2.1e1./1.0e3);dq2.*t8.*(dq5.*t5.*5.0e1-dq3.*t131-dq4.*t131+dq5.*cos(q3+t37).*5.0e1).*(-2.1e1./1.0e3)+dq6.*t4.*t200.*(2.1e1./1.0e3)+dq2.*dq5.*t39.*t131.*(2.1e1./2.0e1);t4.*(t216+dq6.*t9.*t200.*(2.1e1./1.0e1)-t9.*t204.*t207)-t9.*(t217+t218+dq6.*t4.*t200.*(2.1e1./1.0e1))+dq7.*t11.*t215.*(2.1e1./1.0e3);t10.*(dq7.*t11.*t215.*(-2.1e1./1.0e1)+t4.*t204.*t207+dq2.*dq5.*t9.*t130.*(2.1e1./1.0e3))-t11.*(t11.*(t217+t218+dq6.*t211.*(2.1e1./1.0e3))+t10.*(t216+dq6.*t213.*(2.1e1./1.0e3)-t9.*t204.*t207)-dq7.*t10.*t215.*(2.1e1./1.0e1))];
end
if nargout > 4
    t219 = t5.*t8.*1.4164748e7;
    t220 = t6.*t7.*1.4164748e7;
    t221 = t7.*t8.*2.37344e6;
    t222 = t4.*t5.*t6.*1.79145e5;
    t223 = t5.*t8.*t10.*1.42171e5;
    t224 = t6.*t7.*t10.*1.42171e5;
    t225 = t7.*t8.*t9.*4.582e3;
    t226 = t5.*t6.*t9.*t11.*1.42171e5;
    G = [0.0;0.0;g.*(t5.*-4.812199e7-t7.*6.51847e5+t219+t220+t221+t222+t223+t224+t225+t226-t5.*t6.*2.37344e6-t4.*t7.*t8.*1.79145e5-t5.*t6.*t9.*4.582e3-t7.*t8.*t9.*t11.*1.42171e5).*1.0e-7;g.*(t219+t220+t221+t222+t223+t224+t225+t226-t5.*t6.*2.37344e6-t4.*t7.*t8.*1.79145e5-t5.*t6.*t9.*4.582e3-t7.*t8.*t9.*t11.*1.42171e5).*1.0e-7;g.*t130.*(t4.*4.582e3+t9.*1.79145e5-t4.*t11.*1.42171e5).*1.0e-7;g.*(t5.*t6.*t11.*1.42171e5-t7.*t8.*t11.*1.42171e5+t5.*t8.*t9.*t10.*1.42171e5+t6.*t7.*t9.*t10.*1.42171e5).*1.0e-7;0.0];
end
